simulink model "ME_v7_GOOD_1"  (Simulink 7.5)
settings: Solver=ode45  StartTime=0.0  StopTime=10.0  RelTol=1e-3
values from neighbouring files (symbols this model uses):
  R0 = single(Euler2DCMdeg( PHI_IC, THETA_IC, PSI_IC ))    [demoz2SlugsV5.m]
libraries: aerolibconvert2 x1, simulink x1, dspmtrx3 x1
settings Model: Creator=Robert  LastModifiedBy=Robert

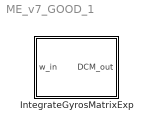
== system ME_v7_GOOD_1 ==
  IntegrateGyrosMatrixExp : Subsystem

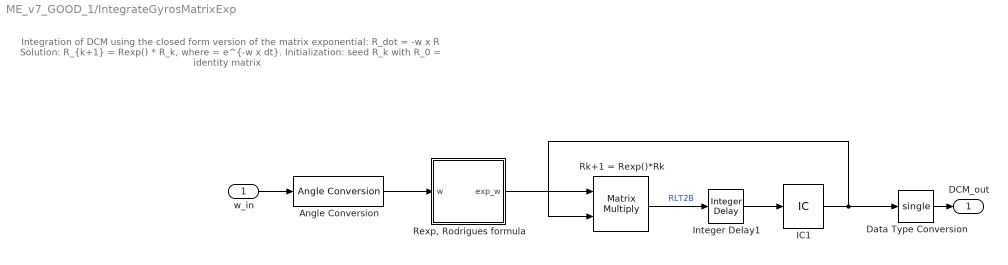
== system ME_v7_GOOD_1/IntegrateGyrosMatrixExp ==
  note: Integration of DCM using the closed form version of the matrix exponential:
      | R_dot = -w x R
      | Solution:  R_{k+1} = Rexp() * R_k, where  = e^{-w x dt}.
      | Initialization:  seed R_k with R_0 = identity matrix
  w_in : Inport
  Angle Conversion : aerolibconvert2/Angle Conversion  SystemSampleTime=-1  IU=deg  OU=rad
  Data Type Conversion : DataTypeConversion  OutDataTypeMode=single  OutDataType=fixdt(1, 16)  OutScaling=2^0  OutDataTypeStr=single
  IC1 : InitialCondition  Value=R0
  Integer Delay1 : simulink/Discrete/Integer Delay  vinit=0.0  samptime=-1  NumDelays=1
  "Rexp, Rodrigues formula" : Subsystem
  Rk+1 = Rexp()*Rk : Product  Multiplication=Matrix(*)  OutDataTypeMode=double  OutDataType=sfix(16)  OutScaling=2^0  OutDataTypeStr=double  RndMeth=Zero
  DCM_out : Outport
  wires:
  w_in/1 -> Angle Conversion/1
  Rk+1 = Rexp()*Rk/1 -> Integer Delay1/1  "RLT2B"
  Data Type Conversion/1 -> DCM_out/1
  IC1/1 -> Data Type Conversion/1, Rk+1 = Rexp()*Rk/2
  Integer Delay1/1 -> IC1/1
  "Rexp, Rodrigues formula"/1(exp_w) -> Rk+1 = Rexp()*Rk/1
  Angle Conversion/1 -> "Rexp, Rodrigues formula"/1(w)

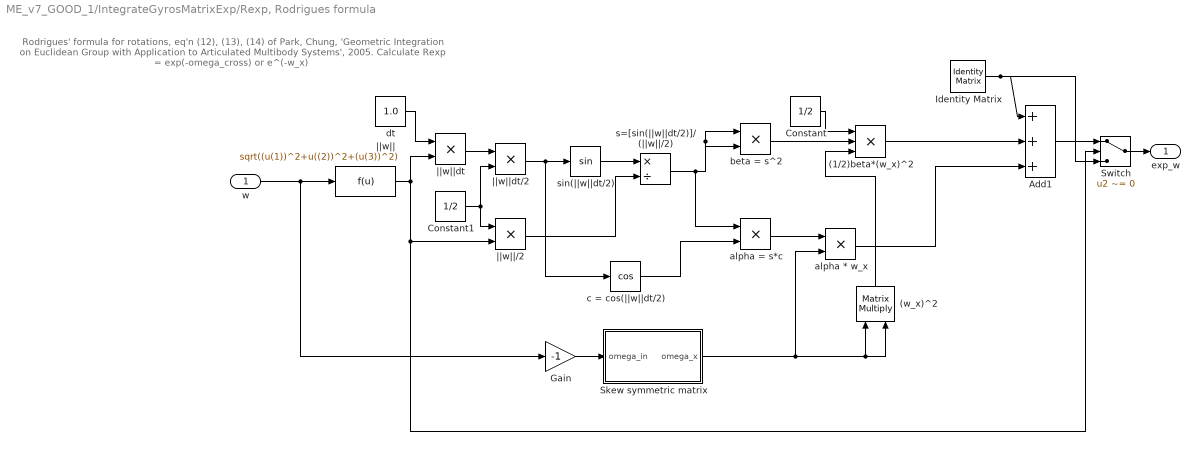
== system ME_v7_GOOD_1/IntegrateGyrosMatrixExp/Rexp, Rodrigues formula ==
  note: Rodrigues' formula for rotations, eq'n (12), (13), (14) of
      | Park, Chung, 'Geometric Integration on Euclidean
      | Group with Application to Articulated Multibody Systems', 2005.
      | Calculate Rexp = exp(-omega_cross) or e^(-w_x)
  w : Inport
  (1/2)beta*(w_x)^2 : Product  Inputs=3  OutDataTypeMode=double  OutDataType=fixdt(1, 16)  OutScaling=2^0  OutDataTypeStr=double  RndMeth=Zero
  (w_x)^2 : Product  Multiplication=Matrix(*)  OutDataTypeMode=double  OutDataType=fixdt(1, 16)  OutScaling=2^0  OutDataTypeStr=double  RndMeth=Zero
  Add1 : Sum  Inputs=+++  AccumDataTypeStr=double  OutDataType=sfix(16)  OutScaling=2^-10
  Constant : Constant  Value=1/2  OutDataTypeMode=double  OutDataType=fixdt(1, 16)  OutScaling=2^0  OutDataTypeStr=double
  Constant1 : Constant  Value=1/2  OutDataTypeMode=double  OutDataType=fixdt(1, 16)  OutScaling=2^0  OutDataTypeStr=double
  Gain : Gain  Gain=-1  ParameterDataType=fixdt(1, 16)  ParameterScaling=2^0  OutDataTypeMode=double  OutDataType=fixdt(1, 16)  OutScaling=2^0  OutDataTypeStr=double
  Identity Matrix : dspmtrx3/Identity Matrix  Inherit=off  N=3  Ts=inf  dataType=double  isSigned=on  wordLen=16  udDataType=sfix(16)  fracBitsMode=Best precision  numFracBits=15
  Skew symmetric matrix : Subsystem
  Switch : Switch  Criteria=u2 ~= 0  OutDataType=fixdt(1, 16)  OutScaling=2^0
  alpha * w_x : Product  OutDataTypeMode=double  OutDataType=fixdt(1, 16)  OutScaling=2^0  OutDataTypeStr=double  RndMeth=Zero
  alpha = s*c : Product  OutDataTypeMode=double  OutDataType=fixdt(1, 16)  OutScaling=2^0  OutDataTypeStr=double  RndMeth=Zero
  beta = s^2 : Product  OutDataTypeMode=double  OutDataType=fixdt(1, 16)  OutScaling=2^0  OutDataTypeStr=double  RndMeth=Zero
  c = cos(||w||dt/2) : Trigonometry  Operator=cos  OutputSignalType=real
  dt : Constant  Value=1.0  OutDataTypeMode=double  OutDataType=fixdt(1, 16)  OutScaling=2^0  OutDataTypeStr=double
  s=[sin(||w||dt/2)]/ (||w||/2) : Product  Inputs=*/  OutDataType=fixdt(1, 16)  OutScaling=2^-10
  sin(||w||dt/2) : Trigonometry  OutputSignalType=real
  ||w|| : Fcn  Expr=sqrt((u(1))^2+u((2))^2+(u(3))^2)
  ||w||/2 : Product  OutDataType=fixdt(1, 16)  OutScaling=2^0  RndMeth=Zero
  "||w||dt " : Product  OutDataType=fixdt(1, 16)  OutScaling=2^0  RndMeth=Zero
  ||w||dt/2 : Product  OutDataType=fixdt(1, 16)  OutScaling=2^0  RndMeth=Zero
  exp_w : Outport
  wires:
  Skew symmetric matrix/1(omega_x) -> (w_x)^2/1, (w_x)^2/2, alpha * w_x/2
  w/1 -> Gain/1, ||w||/1
  Identity Matrix/1 -> Add1/1, Switch/3
  Gain/1 -> Skew symmetric matrix/1(omega_in)
  c = cos(||w||dt/2)/1 -> alpha = s*c/2
  alpha = s*c/1 -> alpha * w_x/1
  alpha * w_x/1 -> Add1/3
  (1/2)beta*(w_x)^2/1 -> Add1/2
  Constant/1 -> (1/2)beta*(w_x)^2/1
  beta = s^2/1 -> (1/2)beta*(w_x)^2/2
  (w_x)^2/1 -> (1/2)beta*(w_x)^2/3
  s=[sin(||w||dt/2)]/ (||w||/2)/1 -> beta = s^2/1, beta = s^2/2, alpha = s*c/1
  dt/1 -> "||w||dt "/1
  ||w||/1 -> "||w||dt "/2, ||w||/2/2, Switch/2
  "||w||dt "/1 -> ||w||dt/2/1
  Constant1/1 -> ||w||dt/2/2, ||w||/2/1
  ||w||dt/2/1 -> sin(||w||dt/2)/1, c = cos(||w||dt/2)/1
  sin(||w||dt/2)/1 -> s=[sin(||w||dt/2)]/ (||w||/2)/1
  ||w||/2/1 -> s=[sin(||w||dt/2)]/ (||w||/2)/2
  Add1/1 -> Switch/1
  Switch/1 -> exp_w/1

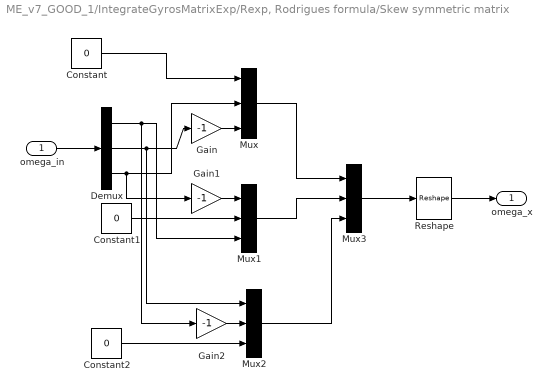
== system ME_v7_GOOD_1/IntegrateGyrosMatrixExp/Rexp, Rodrigues formula/Skew symmetric matrix ==
  omega_in : Inport  OutDataType=fixdt(1, 16)  OutScaling=2^0
  Constant : Constant  Value=0  OutDataType=fixdt(1, 16)  OutScaling=2^0
  Constant1 : Constant  Value=0  OutDataType=fixdt(1, 16)  OutScaling=2^0
  Constant2 : Constant  Value=0  OutDataType=fixdt(1, 16)  OutScaling=2^0
  Demux : Demux  Outputs=3
  Gain : Gain  Gain=-1  ParameterDataType=fixdt(1, 16)  ParameterScaling=2^0  OutDataType=fixdt(1, 16)  OutScaling=2^0
  Gain1 : Gain  Gain=-1  ParameterDataType=fixdt(1, 16)  ParameterScaling=2^0  OutDataType=fixdt(1, 16)  OutScaling=2^0
  Gain2 : Gain  Gain=-1  ParameterDataType=fixdt(1, 16)  ParameterScaling=2^0  OutDataType=fixdt(1, 16)  OutScaling=2^0
  Mux{,1..3} (4 alike) : Mux  Inputs=3
  Reshape : Reshape  OutputDimensionality=Customize  OutputDimensions=[3,3]
  omega_x : Outport  OutDataType=fixdt(1, 16)  OutScaling=2^0
  wires:
  omega_in/1 -> Demux/1
  Reshape/1 -> omega_x/1
  Constant/1 -> Mux/1
  Demux/3 -> Mux/2, Gain1/1
  Demux/2 -> Gain/1, Mux2/1
  Constant1/1 -> Mux1/2
  Demux/1 -> Mux1/3, Gain2/1
  Constant2/1 -> Mux2/3
  Mux/1 -> Mux3/1
  Mux1/1 -> Mux3/2
  Mux2/1 -> Mux3/3
  Mux3/1 -> Reshape/1
  Gain/1 -> Mux/3
  Gain1/1 -> Mux1/1
  Gain2/1 -> Mux2/2
